simulink model "Sistema_Pra_4"  (R2023a)
settings: Solver=ode23t  StartTime=0.0  StopTime=10  MaxStep=1e-3  RelTol=1e-3
libraries: fl_lib x21, nesl_utility x9, slpidlib x2
settings Model: LastModifiedBy=mexic
settings DataIOCC: ReturnWorkspaceOutputs=off  TimeSaveName=t
settings DebuggingCC: AlgebraicLoopMsg=none  ArtificialAlgebraicLoopMsg=none  MaxConsecutiveZCsMsg=none
settings RTWCC: GPUComputeCapability=5.0

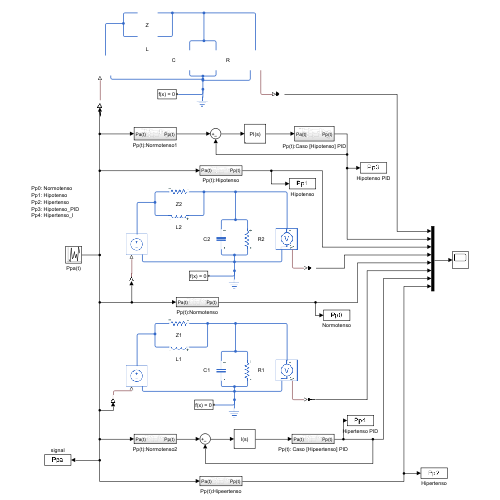
[thumbnail: Simulink's stored preview of the top-level diagram]
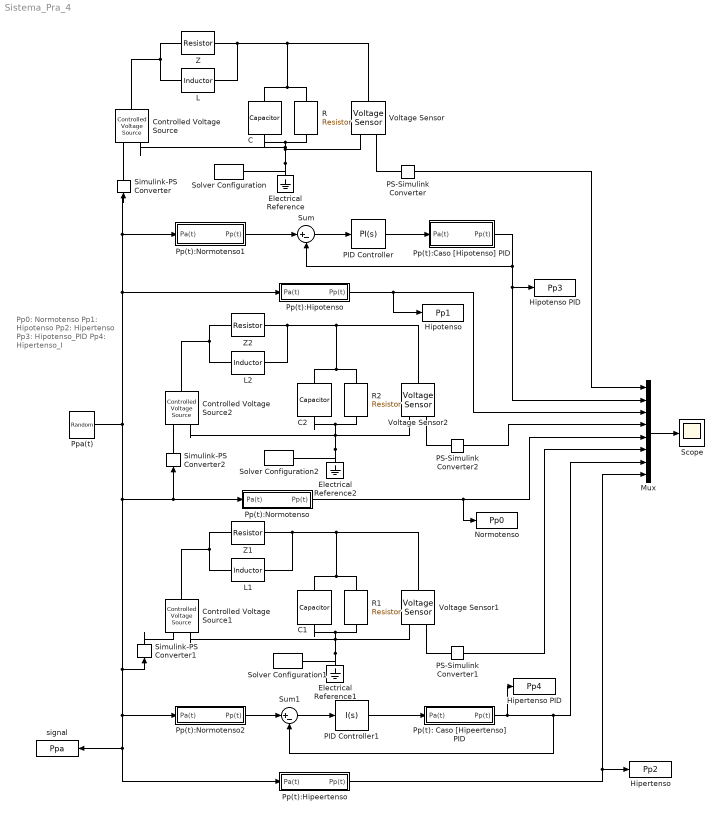
== system Sistema_Pra_4 ==
  note: Pp0: Normotenso
      | Pp1: Hipotenso
      | Pp2: Hipertenso
      | Pp3: Hipotenso_PID
      | Pp4: Hipertenso_I
  C : fl_lib/Electrical/Electrical Elements/Capacitor  c=0.250 F  r=1e-6 Ohm  g=0 1/Ohm  i_specify=off  i_priority=None  i=0 A  i_nominal_specify=off  i_nominal_unit=A  i_nominal_value=1  v_specify=off  v_priority=None  v=0 V  v_nominal_specify=off  v_nominal_unit=V  v_nominal_value=1  vc_specify=off  vc_priority=High  vc=0 V  vc_nominal_specify=off  vc_nominal_unit=V  vc_nominal_value=1
  C1 : fl_lib/Electrical/Electrical Elements/Capacitor  c=2.500 F  r=1e-6 Ohm  g=0 1/Ohm  i_specify=off  i_priority=None  i=0 A  i_nominal_specify=off  i_nominal_unit=A  i_nominal_value=1  v_specify=off  v_priority=None  v=0 V  v_nominal_specify=off  v_nominal_unit=V  v_nominal_value=1  vc_specify=off  vc_priority=High  vc=0 V  vc_nominal_specify=off  vc_nominal_unit=V  vc_nominal_value=1
  C2 : fl_lib/Electrical/Electrical Elements/Capacitor  c=1.500 F  r=1e-6 Ohm  g=0 1/Ohm  i_specify=off  i_priority=None  i=0 A  i_nominal_specify=off  i_nominal_unit=A  i_nominal_value=1  v_specify=off  v_priority=None  v=0 V  v_nominal_specify=off  v_nominal_unit=V  v_nominal_value=1  vc_specify=off  vc_priority=High  vc=0 V  vc_nominal_specify=off  vc_nominal_unit=V  vc_nominal_value=1
  Controlled Voltage Source : fl_lib/Electrical/Electrical Sources/Controlled Voltage Source
  Controlled Voltage Source1 : fl_lib/Electrical/Electrical Sources/Controlled Voltage Source
  Controlled Voltage Source2 : fl_lib/Electrical/Electrical Sources/Controlled Voltage Source
  Electrical Reference : fl_lib/Electrical/Electrical Elements/Electrical Reference
  Electrical Reference1 : fl_lib/Electrical/Electrical Elements/Electrical Reference
  Electrical Reference2 : fl_lib/Electrical/Electrical Elements/Electrical Reference
  Hipertenso : ToWorkspace  VariableName=Pp2  SampleTime=-1
      settings: Save2DSignal=2-D array (concatenate along first dimension)
  Hipertenso PID : ToWorkspace  VariableName=Pp4  SampleTime=-1
      settings: Save2DSignal=2-D array (concatenate along first dimension)
  Hipotenso : ToWorkspace  VariableName=Pp1  SampleTime=-1
      settings: Save2DSignal=2-D array (concatenate along first dimension)
  Hipotenso PID : ToWorkspace  VariableName=Pp3  SampleTime=-1
      settings: Save2DSignal=2-D array (concatenate along first dimension)
  L : fl_lib/Electrical/Electrical Elements/Inductor  l=0.005 H  r=0 Ohm  g=1e-9 1/Ohm  i_specify=off  i_priority=None  i=0 A  i_nominal_specify=off  i_nominal_unit=A  i_nominal_value=1  v_specify=off  v_priority=None  v=0 V  v_nominal_specify=off  v_nominal_unit=V  v_nominal_value=1  i_L_specify=off  i_L_priority=High  i_L=0 A  i_L_nominal_specify=off  i_L_nominal_unit=A  i_L_nominal_value=1
  L1 : fl_lib/Electrical/Electrical Elements/Inductor  l=0.020 H  r=0 Ohm  g=1e-9 1/Ohm  i_specify=off  i_priority=None  i=0 A  i_nominal_specify=off  i_nominal_unit=A  i_nominal_value=1  v_specify=off  v_priority=None  v=0 V  v_nominal_specify=off  v_nominal_unit=V  v_nominal_value=1  i_L_specify=off  i_L_priority=High  i_L=0 A  i_L_nominal_specify=off  i_L_nominal_unit=A  i_L_nominal_value=1
  L2 : fl_lib/Electrical/Electrical Elements/Inductor  l=0.010 H  r=0 Ohm  g=1e-9 1/Ohm  i_specify=off  i_priority=None  i=0 A  i_nominal_specify=off  i_nominal_unit=A  i_nominal_value=1  v_specify=off  v_priority=None  v=0 V  v_nominal_specify=off  v_nominal_unit=V  v_nominal_value=1  i_L_specify=off  i_L_priority=High  i_L=0 A  i_L_nominal_specify=off  i_L_nominal_unit=A  i_L_nominal_value=1
  Mux : Mux  Inputs=8
  Normotenso : ToWorkspace  VariableName=Pp0  SampleTime=-1
      settings: Save2DSignal=2-D array (concatenate along first dimension)
  PID Controller : slpidlib/PID Controller  Controller=PI  Form=Parallel  TimeDomain=Continuous-time  UseExternalTs=off  SampleTime=-1  IntegratorMethod=Forward Euler  FilterMethod=Forward Euler  ControllerParametersSource=internal  P=4.21636346738391e-05  I=3267.68674685278  UseKiTs=off  D=0  N=100  UseFilter=on  TunerSelectOption=Transfer Function Based (PID Tuner App)  InitialConditionSource=internal  InitialConditionForIntegrator=0  InitialConditionForFilter=0  DifferentiatorICPrevScaledInput=0  ExternalReset=none  TrackingMode=off  Kt=1  LimitOutput=off  SatLimitsSource=internal  UpperSaturationLimit=inf  LowerSaturationLimit=-inf  LinearizeAsGain=on  AntiWindupMode=none  Kb=1  LimitIntegrator=off  UpperIntegratorSaturationLimit=inf  LowerIntegratorSaturationLimit=-inf  POutMin=[]  POutMax=[]  IOutMin=[]  IOutMax=[]  DOutMin=[]  DOutMax=[]  NOutMin=[]  NOutMax=[]  SumOutMin=[]  SumOutMax=[]  SaturationOutMin=[]  SaturationOutMax=[]  PParamMin=[]  PParamMax=[]  IParamMin=[]  IParamMax=[]  DParamMin=[]  DParamMax=[]  NParamMin=[]  NParamMax=[]  KbParamMin=[]  KbParamMax=[]  KtParamMin=[]  KtParamMax=[]  KbOutMin=[]  KbOutMax=[]  KtOutMin=[]  KtOutMax=[]  IntegratorOutMin=[]  IntegratorOutMax=[]  FilterOutMin=[]  FilterOutMax=[]  SumI1OutMin=[]  SumI1OutMax=[]  SumI2OutMin=[]  SumI2OutMax=[]  SumI3OutMin=[]  SumI3OutMax=[]  SumI4OutMin=[]  SumI4OutMax=[]  SumDOutMin=[]  SumDOutMax=[]  DifferentiatorOutMin=[]  DifferentiatorOutMax=[]  FilterDiffOutCoefMin=[]  FilterDiffOutCoefMax=[]  ReciprocalOutMin=[]  ReciprocalOutMax=[]  SumDenOutMin=[]  SumDenOutMax=[]  SumNumOutMin=[]  SumNumOutMax=[]  DivideOutMin=[]  DivideOutMax=[]  UdiffTsProdOutMin=[]  UdiffTsProdOutMax=[]  NTsProdOutMin=[]  NTsProdOutMax=[]  UintegralTsProdOutMin=[]  UintegralTsProdOutMax=[]  UngainTsProdOutMin=[]  UngainTsProdOutMax=[]  ClampingZeroOutDataTypeStr=Inherit: Inherit via back propagation  ClampingZeroOutMin=[]  ClampingZeroOutMax=[]  FilterDenConstantOutDataTypeStr=Inherit: Inherit via back propagation  FilterDenConstantOutMin=[]  FilterDenConstantOutMax=[]  PCopyOutDataTypeStr=Inherit: Inherit via back propagation  PCopyOutMin=[]  PCopyOutMax=[]  NCopyOutDataTypeStr=Inherit: Inherit via back propagation  NCopyOutMin=[]  NCopyOutMax=[]  IntegratorContinuousStateAttributes=''  IntegratorStateMustResolveToSignalObject=off  IntegratorRTWStateStorageClass=Auto  FilterContinuousStateAttributes=''  FilterStateMustResolveToSignalObject=off  FilterRTWStateStorageClass=Auto  ParallelPVariant=InternalParameters  IdealPVariant=Disabled  IVariant=InternalParameters  DVariant=Disabled  IntegratorVariant=Continuous  SatVariant=Disabled  AWVariant=Passthrough  PCopyVariant=Disabled  TRVariant=Disabled  FdbkBlocksVariant=Forward  IdealPFdbkVariant=Disabled  SatFdbkVariant=Disabled  DerivativeFilterVariant=Disabled  NVariant=Disabled  NCopyVariant=Disabled_SignalSpec  FilterICVariant=Disabled  IntegratorICVariant=InternalICs  ExternalResetVariant=Disabled  TRSumVariant=Passthrough  SumFdbkVariant=Disabled  SumVariant=Sum_PI  TsampFilterVariant=InternalTs  TsampNgainVariant=Passthrough  TsampIntegralVariant=Disabled_SignalSpec  ExternalSaturationOutDataTypeStr=Inherit: Same as second input
  PID Controller1 : slpidlib/PID Controller  Controller=I  Form=Ideal  TimeDomain=Continuous-time  UseExternalTs=off  SampleTime=-1  IntegratorMethod=Forward Euler  FilterMethod=Forward Euler  ControllerParametersSource=internal  P=0.00010357142839881  I=31622776.4962745  UseKiTs=off  D=0  N=100  UseFilter=on  TunerSelectOption=Transfer Function Based (PID Tuner App)  InitialConditionSource=internal  InitialConditionForIntegrator=0  InitialConditionForFilter=0  DifferentiatorICPrevScaledInput=0  ExternalReset=none  TrackingMode=off  Kt=1  LimitOutput=off  SatLimitsSource=internal  UpperSaturationLimit=inf  LowerSaturationLimit=-inf  LinearizeAsGain=on  AntiWindupMode=none  Kb=1  LimitIntegrator=off  UpperIntegratorSaturationLimit=inf  LowerIntegratorSaturationLimit=-inf  POutMin=[]  POutMax=[]  IOutMin=[]  IOutMax=[]  DOutMin=[]  DOutMax=[]  NOutMin=[]  NOutMax=[]  SumOutMin=[]  SumOutMax=[]  SaturationOutMin=[]  SaturationOutMax=[]  PParamMin=[]  PParamMax=[]  IParamMin=[]  IParamMax=[]  DParamMin=[]  DParamMax=[]  NParamMin=[]  NParamMax=[]  KbParamMin=[]  KbParamMax=[]  KtParamMin=[]  KtParamMax=[]  KbOutMin=[]  KbOutMax=[]  KtOutMin=[]  KtOutMax=[]  IntegratorOutMin=[]  IntegratorOutMax=[]  FilterOutMin=[]  FilterOutMax=[]  SumI1OutMin=[]  SumI1OutMax=[]  SumI2OutMin=[]  SumI2OutMax=[]  SumI3OutMin=[]  SumI3OutMax=[]  SumI4OutMin=[]  SumI4OutMax=[]  SumDOutMin=[]  SumDOutMax=[]  DifferentiatorOutMin=[]  DifferentiatorOutMax=[]  FilterDiffOutCoefMin=[]  FilterDiffOutCoefMax=[]  ReciprocalOutMin=[]  ReciprocalOutMax=[]  SumDenOutMin=[]  SumDenOutMax=[]  SumNumOutMin=[]  SumNumOutMax=[]  DivideOutMin=[]  DivideOutMax=[]  UdiffTsProdOutMin=[]  UdiffTsProdOutMax=[]  NTsProdOutMin=[]  NTsProdOutMax=[]  UintegralTsProdOutMin=[]  UintegralTsProdOutMax=[]  UngainTsProdOutMin=[]  UngainTsProdOutMax=[]  ClampingZeroOutDataTypeStr=Inherit: Inherit via back propagation  ClampingZeroOutMin=[]  ClampingZeroOutMax=[]  FilterDenConstantOutDataTypeStr=Inherit: Inherit via back propagation  FilterDenConstantOutMin=[]  FilterDenConstantOutMax=[]  PCopyOutDataTypeStr=Inherit: Inherit via back propagation  PCopyOutMin=[]  PCopyOutMax=[]  NCopyOutDataTypeStr=Inherit: Inherit via back propagation  NCopyOutMin=[]  NCopyOutMax=[]  IntegratorContinuousStateAttributes=''  IntegratorStateMustResolveToSignalObject=off  IntegratorRTWStateStorageClass=Auto  FilterContinuousStateAttributes=''  FilterStateMustResolveToSignalObject=off  FilterRTWStateStorageClass=Auto  ParallelPVariant=Disabled  IdealPVariant=Disabled  IVariant=InternalParameters  DVariant=Disabled  IntegratorVariant=Continuous  SatVariant=Disabled  AWVariant=Passthrough  PCopyVariant=Disabled  TRVariant=Disabled  FdbkBlocksVariant=Forward  IdealPFdbkVariant=Disabled  SatFdbkVariant=Disabled  DerivativeFilterVariant=Disabled  NVariant=Disabled  NCopyVariant=Disabled_SignalSpec  FilterICVariant=Disabled  IntegratorICVariant=InternalICs  ExternalResetVariant=Disabled  TRSumVariant=Passthrough  SumFdbkVariant=Disabled  SumVariant=Passthrough_I  TsampFilterVariant=InternalTs  TsampNgainVariant=Passthrough  TsampIntegralVariant=Disabled_SignalSpec  ExternalSaturationOutDataTypeStr=Inherit: Same as second input
  PS-Simulink Converter : nesl_utility/PS-Simulink Converter  PhysicalDomain=network_engine_domain  SubClassName=ps_output  LeftPortType=input  RightPortType=output  PseudoPeriodic=off  Frequencies=[]  VectorFormat=inherit  Unit=inherit  AffineConversion=off
  PS-Simulink Converter1 : nesl_utility/PS-Simulink Converter  PhysicalDomain=network_engine_domain  SubClassName=ps_output  LeftPortType=input  RightPortType=output  PseudoPeriodic=off  Frequencies=[]  VectorFormat=inherit  Unit=inherit  AffineConversion=off
  PS-Simulink Converter2 : nesl_utility/PS-Simulink Converter  PhysicalDomain=network_engine_domain  SubClassName=ps_output  LeftPortType=input  RightPortType=output  PseudoPeriodic=off  Frequencies=[]  VectorFormat=inherit  Unit=inherit  AffineConversion=off
  Pp(t): Caso [Hipeertenso] PID : Subsystem
  Pp(t):Caso [Hipotenso] PID : Subsystem
  Pp(t):Hipeertenso : Subsystem
  Pp(t):Hipotenso : Subsystem
  Pp(t):Normotenso : Subsystem
  Pp(t):Normotenso1 : Subsystem
  Pp(t):Normotenso2 : Subsystem
  Ppa(t) : UniformRandomNumber  Minimum=-0.2  Seed=106  SampleTime=0.5
  R : fl_lib/Electrical/Electrical Elements/Resistor  R=0.600 Ohm  i_specify=off  i_priority=None  i=0 A  i_nominal_specify=off  i_nominal_unit=A  i_nominal_value=1  v_specify=off  v_priority=None  v=0 V  v_nominal_specify=off  v_nominal_unit=V  v_nominal_value=1
  R1 : fl_lib/Electrical/Electrical Elements/Resistor  R=1.400 Ohm  i_specify=off  i_priority=None  i=0 A  i_nominal_specify=off  i_nominal_unit=A  i_nominal_value=1  v_specify=off  v_priority=None  v=0 V  v_nominal_specify=off  v_nominal_unit=V  v_nominal_value=1
  R2 : fl_lib/Electrical/Electrical Elements/Resistor  R=0.950 Ohm  i_specify=off  i_priority=None  i=0 A  i_nominal_specify=off  i_nominal_unit=A  i_nominal_value=1  v_specify=off  v_priority=None  v=0 V  v_nominal_specify=off  v_nominal_unit=V  v_nominal_value=1
  Scope : Scope
  Simulink-PS Converter : nesl_utility/Simulink-PS Converter  PhysicalDomain=network_engine_domain  SubClassName=ps_input  LeftPortType=input  RightPortType=output  PseudoPeriodic=off  Frequencies=[]  NoiseDistribution=none  NoiseParameters=[]  Unit=1  AffineConversion=off  FilteringAndDerivatives=provide  SimscapeFilterOrder=1  InputFilterTimeConstant=0.001  UdotUserProvided=0
  Simulink-PS Converter1 : nesl_utility/Simulink-PS Converter  PhysicalDomain=network_engine_domain  SubClassName=ps_input  LeftPortType=input  RightPortType=output  PseudoPeriodic=off  Frequencies=[]  NoiseDistribution=none  NoiseParameters=[]  Unit=1  AffineConversion=off  FilteringAndDerivatives=provide  SimscapeFilterOrder=1  InputFilterTimeConstant=0.001  UdotUserProvided=0
  Simulink-PS Converter2 : nesl_utility/Simulink-PS Converter  PhysicalDomain=network_engine_domain  SubClassName=ps_input  LeftPortType=input  RightPortType=output  PseudoPeriodic=off  Frequencies=[]  NoiseDistribution=none  NoiseParameters=[]  Unit=1  AffineConversion=off  FilteringAndDerivatives=provide  SimscapeFilterOrder=1  InputFilterTimeConstant=0.001  UdotUserProvided=0
  Solver Configuration : nesl_utility/Solver Configuration  PhysicalDomain=network_engine_domain  SubClassName=solver  LeftPortType=input  RightPortType=generic  Tones=[]  Harmonics=[]  SimulateNoise=off  Profile=off  UseLocalSampling=off  EnableSwitchedLinearOptims=on  FrequencyDomain=off  UseCCode=off  RelTol=0.001  AbsTol=0.001  MinStep=1e-09  ToWorkspace=off  RevertToSquareIcSolve=off  NumHomotopyIterations=100  PhasorMode=off  PhasorModeNumHarmonics=1  ConsistencySolver=NEWTON_XTOL_AFTER_FTOL  IndexReductionMethod=DerivativeReplacement  DoDC=off  ResidualTolerance=1e-09  ConsistencyTolSource=GLOBAL  ConsistencyAbsTol=0.001  ConsistencyRelTol=0.001  ConsistencyTolFactor=0.001  UseLocalSolver=off  LocalSolverChoice=NE_BACKWARD_EULER_ADVANCER  ResolveIndetEquations=on  FunctionEvalNumThread=1  LocalSolverSampleTime=0.001  DoFixedCost=off  MaxNonlinIter=3  MaxModeIter=2  ComputeImpulses=off  ImpulseIterations=2  LinearAlgebra=auto  LinearAlgebraNumThread=0  EquationFormulation=NE_TIME_EF  DelaysMemoryBudget=1024  AutomaticFiltering=on  FilteringTimeConstant=0.001  PartitionStorageMethod=AS_NEEDED  PartitionMemoryBudget=1024  PartitionMethod=ROBUST
  Solver Configuration1 : nesl_utility/Solver Configuration  PhysicalDomain=network_engine_domain  SubClassName=solver  LeftPortType=input  RightPortType=generic  Tones=[]  Harmonics=[]  SimulateNoise=off  Profile=off  UseLocalSampling=off  EnableSwitchedLinearOptims=on  FrequencyDomain=off  UseCCode=off  RelTol=0.001  AbsTol=0.001  MinStep=1e-09  ToWorkspace=off  RevertToSquareIcSolve=off  NumHomotopyIterations=100  PhasorMode=off  PhasorModeNumHarmonics=1  ConsistencySolver=NEWTON_XTOL_AFTER_FTOL  IndexReductionMethod=DerivativeReplacement  DoDC=off  ResidualTolerance=1e-09  ConsistencyTolSource=GLOBAL  ConsistencyAbsTol=0.001  ConsistencyRelTol=0.001  ConsistencyTolFactor=0.001  UseLocalSolver=off  LocalSolverChoice=NE_BACKWARD_EULER_ADVANCER  ResolveIndetEquations=on  FunctionEvalNumThread=1  LocalSolverSampleTime=0.001  DoFixedCost=off  MaxNonlinIter=3  MaxModeIter=2  ComputeImpulses=off  ImpulseIterations=2  LinearAlgebra=auto  LinearAlgebraNumThread=0  EquationFormulation=NE_TIME_EF  DelaysMemoryBudget=1024  AutomaticFiltering=on  FilteringTimeConstant=0.001  PartitionStorageMethod=AS_NEEDED  PartitionMemoryBudget=1024  PartitionMethod=ROBUST
  Solver Configuration2 : nesl_utility/Solver Configuration  PhysicalDomain=network_engine_domain  SubClassName=solver  LeftPortType=input  RightPortType=generic  Tones=[]  Harmonics=[]  SimulateNoise=off  Profile=off  UseLocalSampling=off  EnableSwitchedLinearOptims=on  FrequencyDomain=off  UseCCode=off  RelTol=0.001  AbsTol=0.001  MinStep=1e-09  ToWorkspace=off  RevertToSquareIcSolve=off  NumHomotopyIterations=100  PhasorMode=off  PhasorModeNumHarmonics=1  ConsistencySolver=NEWTON_XTOL_AFTER_FTOL  IndexReductionMethod=DerivativeReplacement  DoDC=off  ResidualTolerance=1e-09  ConsistencyTolSource=GLOBAL  ConsistencyAbsTol=0.001  ConsistencyRelTol=0.001  ConsistencyTolFactor=0.001  UseLocalSolver=off  LocalSolverChoice=NE_BACKWARD_EULER_ADVANCER  ResolveIndetEquations=on  FunctionEvalNumThread=1  LocalSolverSampleTime=0.001  DoFixedCost=off  MaxNonlinIter=3  MaxModeIter=2  ComputeImpulses=off  ImpulseIterations=2  LinearAlgebra=auto  LinearAlgebraNumThread=0  EquationFormulation=NE_TIME_EF  DelaysMemoryBudget=1024  AutomaticFiltering=on  FilteringTimeConstant=0.001  PartitionStorageMethod=AS_NEEDED  PartitionMemoryBudget=1024  PartitionMethod=ROBUST
  Sum : Sum  Inputs=|+-
  Sum1 : Sum  Inputs=|+-
  Voltage Sensor : fl_lib/Electrical/Electrical Sensors/Voltage Sensor
  Voltage Sensor1 : fl_lib/Electrical/Electrical Sensors/Voltage Sensor
  Voltage Sensor2 : fl_lib/Electrical/Electrical Sensors/Voltage Sensor
  Z : fl_lib/Electrical/Electrical Elements/Resistor  R=0.020 Ohm  i_specify=off  i_priority=None  i=0 A  i_nominal_specify=off  i_nominal_unit=A  i_nominal_value=1  v_specify=off  v_priority=None  v=0 V  v_nominal_specify=off  v_nominal_unit=V  v_nominal_value=1
  Z1 : fl_lib/Electrical/Electrical Elements/Resistor  R=0.050 Ohm  i_specify=off  i_priority=None  i=0 A  i_nominal_specify=off  i_nominal_unit=A  i_nominal_value=1  v_specify=off  v_priority=None  v=0 V  v_nominal_specify=off  v_nominal_unit=V  v_nominal_value=1
  Z2 : fl_lib/Electrical/Electrical Elements/Resistor  R=0.033 Ohm  i_specify=off  i_priority=None  i=0 A  i_nominal_specify=off  i_nominal_unit=A  i_nominal_value=1  v_specify=off  v_priority=None  v=0 V  v_nominal_specify=off  v_nominal_unit=V  v_nominal_value=1
  signal : ToWorkspace  VariableName=Ppa  SampleTime=-1
      settings: Save2DSignal=2-D array (concatenate along first dimension)
  wires:
  Mux/1 -> Scope/1
  Ppa(t)/1 -> Pp(t):Hipotenso/1(Pa(t)), Pp(t):Normotenso1/1(Pa(t)), Simulink-PS Converter/1, Pp(t):Normotenso/1(Pa(t)), Simulink-PS Converter2/1, Simulink-PS Converter1/1, signal/1, Pp(t):Hipeertenso/1(Pa(t)), Pp(t):Normotenso2/1(Pa(t))
  Pp(t):Hipeertenso/1(Pp(t)) -> Mux/8, Hipertenso/1
  Pp(t):Normotenso/1(Pp(t)) -> Normotenso/1, Mux/5
  Pp(t):Hipotenso/1(Pp(t)) -> Hipotenso/1, Mux/3
  PS-Simulink Converter/1 -> Mux/1
  PS-Simulink Converter1/1 -> Mux/6
  PS-Simulink Converter2/1 -> Mux/4
  PID Controller/1 -> Pp(t):Caso [Hipotenso] PID/1(Pa(t))
  Pp(t):Caso [Hipotenso] PID/1(Pp(t)) -> Mux/2, Hipotenso PID/1, Sum/2
  Pp(t):Normotenso1/1(Pp(t)) -> Sum/1
  Sum/1 -> PID Controller/1
  Sum1/1 -> PID Controller1/1
  Pp(t): Caso [Hipeertenso] PID/1(Pp(t)) -> Hipertenso PID/1, Sum1/2, Mux/7
  PID Controller1/1 -> Pp(t): Caso [Hipeertenso] PID/1(Pa(t))
  Pp(t):Normotenso2/1(Pp(t)) -> Sum1/1
  connections:
  Z/RConn1 -- Voltage Sensor/LConn1 -- R/LConn1 -- C/LConn1 -- L/LConn1
  Z/LConn1 -- L/RConn1 -- Controlled Voltage Source/LConn1
  Voltage Sensor/RConn1 -- PS-Simulink Converter/LConn1
  Simulink-PS Converter/RConn1 -- Controlled Voltage Source/RConn1
  C/RConn1 -- Solver Configuration/RConn1 -- Electrical Reference/LConn1 -- Voltage Sensor/RConn2 -- Controlled Voltage Source/RConn2 -- R/RConn1
  Controlled Voltage Source1/LConn1 -- Z1/LConn1 -- L1/RConn1
  C1/LConn1 -- R1/LConn1 -- Z1/RConn1 -- L1/LConn1 -- Voltage Sensor1/LConn1
  Electrical Reference1/LConn1 -- Solver Configuration1/RConn1 -- Controlled Voltage Source1/RConn2 -- Voltage Sensor1/RConn2 -- C1/RConn1 -- R1/RConn1
  Simulink-PS Converter1/RConn1 -- Controlled Voltage Source1/RConn1
  Voltage Sensor1/RConn1 -- PS-Simulink Converter1/LConn1
  Controlled Voltage Source2/LConn1 -- Z2/LConn1 -- L2/RConn1
  C2/LConn1 -- R2/LConn1 -- L2/LConn1 -- Z2/RConn1 -- Voltage Sensor2/LConn1
  Electrical Reference2/LConn1 -- Solver Configuration2/RConn1 -- Voltage Sensor2/RConn2 -- Controlled Voltage Source2/RConn2 -- C2/RConn1 -- R2/RConn1
  Simulink-PS Converter2/RConn1 -- Controlled Voltage Source2/RConn1
  Voltage Sensor2/RConn1 -- PS-Simulink Converter2/LConn1

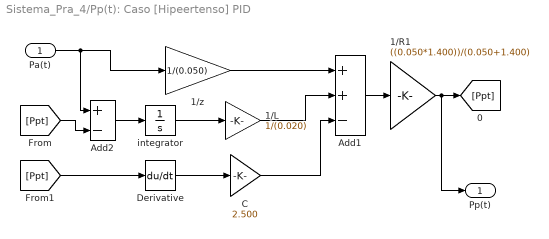
== system Sistema_Pra_4/Pp(t): Caso [Hipeertenso] PID ==
  Pa(t) : Inport
  1/L : Gain  Gain=1/(0.020)
  1/R1 : Gain  Gain=((0.050*1.400))/(0.050+1.400)
  1/z : Gain  Gain=1/(0.050)
  Add1 : Sum  Inputs=++-
  Add2 : Sum  Inputs=+-
  C : Gain  Gain=2.500
  Derivative : Derivative
  integrator : Integrator
  Pp(t) : Outport
  wires:
  1/R1/1 -> Pp(t)/1, [Ppt]
  1/z/1 -> Add1/1
  Pa(t)/1 -> Add2/1, 1/z/1
  integrator/1 -> 1/L/1
  1/L/1 -> Add1/2
  C/1 -> Add1/3
  Add2/1 -> integrator/1
  [Ppt] -> Add2/2
  Derivative/1 -> C/1
  [Ppt] -> Derivative/1
  Add1/1 -> 1/R1/1

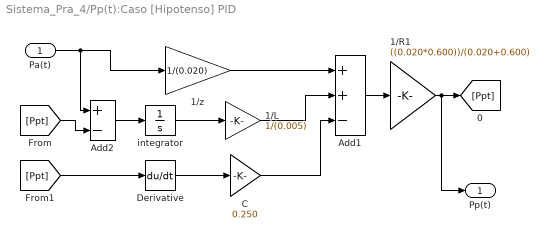
== system Sistema_Pra_4/Pp(t):Caso [Hipotenso] PID ==
  Pa(t) : Inport
  1/L : Gain  Gain=1/(0.005)
  1/R1 : Gain  Gain=((0.020*0.600))/(0.020+0.600)
  1/z : Gain  Gain=1/(0.020)
  Add1 : Sum  Inputs=++-
  Add2 : Sum  Inputs=+-
  C : Gain  Gain=0.250
  Derivative : Derivative
  integrator : Integrator
  Pp(t) : Outport
  wires:
  1/R1/1 -> Pp(t)/1, [Ppt]
  1/z/1 -> Add1/1
  Pa(t)/1 -> Add2/1, 1/z/1
  integrator/1 -> 1/L/1
  1/L/1 -> Add1/2
  C/1 -> Add1/3
  Add2/1 -> integrator/1
  [Ppt] -> Add2/2
  Derivative/1 -> C/1
  [Ppt] -> Derivative/1
  Add1/1 -> 1/R1/1

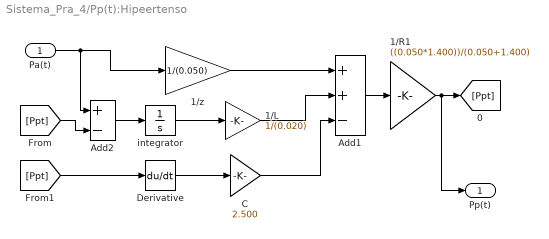
== system Sistema_Pra_4/Pp(t):Hipeertenso ==
  Pa(t) : Inport
  1/L : Gain  Gain=1/(0.020)
  1/R1 : Gain  Gain=((0.050*1.400))/(0.050+1.400)
  1/z : Gain  Gain=1/(0.050)
  Add1 : Sum  Inputs=++-
  Add2 : Sum  Inputs=+-
  C : Gain  Gain=2.500
  Derivative : Derivative
  integrator : Integrator
  Pp(t) : Outport
  wires:
  1/R1/1 -> Pp(t)/1, [Ppt]
  1/z/1 -> Add1/1
  Pa(t)/1 -> Add2/1, 1/z/1
  integrator/1 -> 1/L/1
  1/L/1 -> Add1/2
  C/1 -> Add1/3
  Add2/1 -> integrator/1
  [Ppt] -> Add2/2
  Derivative/1 -> C/1
  [Ppt] -> Derivative/1
  Add1/1 -> 1/R1/1

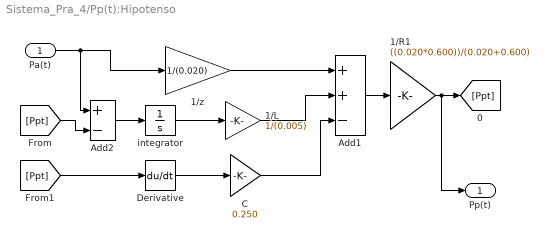
== system Sistema_Pra_4/Pp(t):Hipotenso ==
  Pa(t) : Inport
  1/L : Gain  Gain=1/(0.005)
  1/R1 : Gain  Gain=((0.020*0.600))/(0.020+0.600)
  1/z : Gain  Gain=1/(0.020)
  Add1 : Sum  Inputs=++-
  Add2 : Sum  Inputs=+-
  C : Gain  Gain=0.250
  Derivative : Derivative
  integrator : Integrator
  Pp(t) : Outport
  wires:
  1/R1/1 -> Pp(t)/1, [Ppt]
  1/z/1 -> Add1/1
  Pa(t)/1 -> Add2/1, 1/z/1
  integrator/1 -> 1/L/1
  1/L/1 -> Add1/2
  C/1 -> Add1/3
  Add2/1 -> integrator/1
  [Ppt] -> Add2/2
  Derivative/1 -> C/1
  [Ppt] -> Derivative/1
  Add1/1 -> 1/R1/1

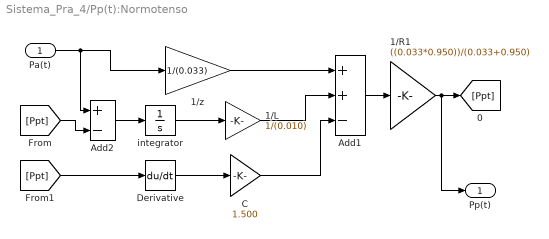
== system Sistema_Pra_4/Pp(t):Normotenso ==
  Pa(t) : Inport
  1/L : Gain  Gain=1/(0.010)
  1/R1 : Gain  Gain=((0.033*0.950))/(0.033+0.950)
  1/z : Gain  Gain=1/(0.033)
  Add1 : Sum  Inputs=++-
  Add2 : Sum  Inputs=+-
  C : Gain  Gain=1.500
  Derivative : Derivative
  integrator : Integrator
  Pp(t) : Outport
  wires:
  1/R1/1 -> Pp(t)/1, [Ppt]
  1/z/1 -> Add1/1
  Pa(t)/1 -> Add2/1, 1/z/1
  integrator/1 -> 1/L/1
  1/L/1 -> Add1/2
  C/1 -> Add1/3
  Add2/1 -> integrator/1
  [Ppt] -> Add2/2
  Derivative/1 -> C/1
  [Ppt] -> Derivative/1
  Add1/1 -> 1/R1/1

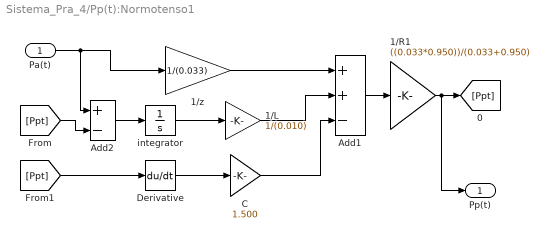
== system Sistema_Pra_4/Pp(t):Normotenso1 ==
  Pa(t) : Inport
  1/L : Gain  Gain=1/(0.010)
  1/R1 : Gain  Gain=((0.033*0.950))/(0.033+0.950)
  1/z : Gain  Gain=1/(0.033)
  Add1 : Sum  Inputs=++-
  Add2 : Sum  Inputs=+-
  C : Gain  Gain=1.500
  Derivative : Derivative
  integrator : Integrator
  Pp(t) : Outport
  wires:
  1/R1/1 -> Pp(t)/1, [Ppt]
  1/z/1 -> Add1/1
  Pa(t)/1 -> Add2/1, 1/z/1
  integrator/1 -> 1/L/1
  1/L/1 -> Add1/2
  C/1 -> Add1/3
  Add2/1 -> integrator/1
  [Ppt] -> Add2/2
  Derivative/1 -> C/1
  [Ppt] -> Derivative/1
  Add1/1 -> 1/R1/1

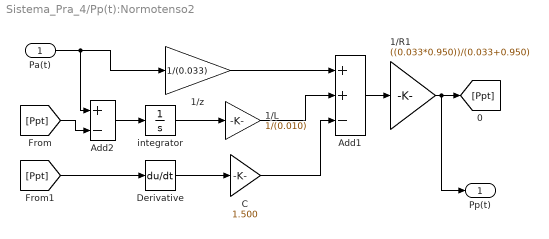
== system Sistema_Pra_4/Pp(t):Normotenso2 ==
  Pa(t) : Inport
  1/L : Gain  Gain=1/(0.010)
  1/R1 : Gain  Gain=((0.033*0.950))/(0.033+0.950)
  1/z : Gain  Gain=1/(0.033)
  Add1 : Sum  Inputs=++-
  Add2 : Sum  Inputs=+-
  C : Gain  Gain=1.500
  Derivative : Derivative
  integrator : Integrator
  Pp(t) : Outport
  wires:
  1/R1/1 -> Pp(t)/1, [Ppt]
  1/z/1 -> Add1/1
  Pa(t)/1 -> Add2/1, 1/z/1
  integrator/1 -> 1/L/1
  1/L/1 -> Add1/2
  C/1 -> Add1/3
  Add2/1 -> integrator/1
  [Ppt] -> Add2/2
  Derivative/1 -> C/1
  [Ppt] -> Derivative/1
  Add1/1 -> 1/R1/1
